simulink model "Bdot_control"  (R2023a)
settings: Solver=ode45  StartTime=0.0  StopTime=5830.0  RelTol=1e-3  EnableMultiTasking=on
libraries: aausat3_lib x6
settings Model: Creator=kasperv  LastModifiedBy=jacobel-omar
settings SolverCC: AlgebraicLoopSolver=TrustRegion
settings DataIOCC: LimitDataPoints=on  SaveFormat=Array  SignalLoggingSaveFormat=ModelDataLogs  ReturnWorkspaceOutputs=off
settings OptimizationCC: ExpressionDepthLimit=2147483647  LifeSpan=inf
settings DebuggingCC: UnderspecifiedInitializationDetection=Classic  MergeDetectMultiDrivingBlocksExec=none  SolverPrmCheckMsg=warning  FcnCallInpInsideContextMsg=warning  UnconnectedInputMsg=warning  UnconnectedOutputMsg=warning  UnconnectedLineMsg=warning  StateNameClashWarn=warning  SFUnexpectedBacktrackingDiag=warning  SFNoUnconditionalDefaultTransitionDiag=warning  SFExecutionAtInitializationDiag=none  ArithmeticOperatorsInVariantConditions=warning
settings HardwareCC: ProdBitPerPointer=32  ProdBitPerSizeT=32  ProdBitPerPtrDiffT=32  ProdLargestAtomicFloat=None  ProdIntDivRoundTo=Undefined  ProdEndianess=Unspecified  ProdWordSize=32  ProdHWDeviceType=32-bit Generic
settings ModelReferenceCC: EnableRefExpFcnMdlSchedulingChecks=on  PropagateSignalLabelsOutOfModel=off
settings SFSimCC: SimUseLocalCustomCode=off  CustomCodeUndefinedFunction=UseInterfaceOnly
settings RTWCC: RTWUseLocalCustomCode=off
settings CodeAppCC: StateflowObjectComments=on
settings GRTTargetCC: TargetLangStandard=C89/C90 (ANSI)  CombineOutputUpdateFcns=off  GRTInterface=on
settings ConfigComp: CovMetricSettings=dw  CovSaveCumulativeToWorkspaceVar=on  CovSaveSingleToWorkspaceVar=on  CovExternalEMLEnable=off

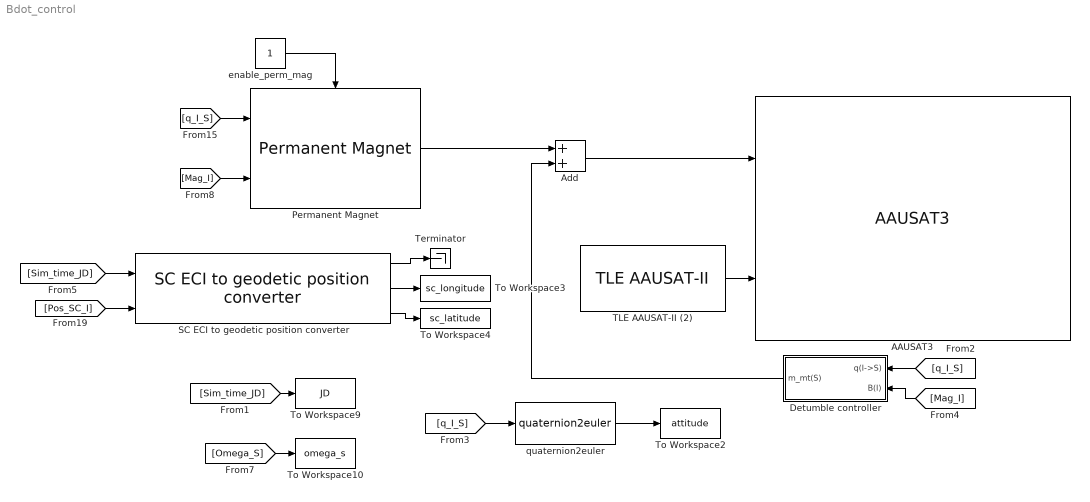
== system Bdot_control ==
  AAUSAT3 : aausat3_lib/AAUSAT3  r_com_s=[0.0493,0.0972,0.0549]  sat_temp_start=293.15  mass_sc=0.7924  Dim=[0.1,0.2,0.1]  inertia_c=[0.001653238447870,0.003461850559345,0.003630565819922]  init_jd=0  q_s_c=|  q_init_I_S=[0 0 0 1]  w_init_s=[0.17,0.17,0.17]  Cd=2  rho=5e-14  solar_m_flux=4.5565e-6  solar_absorb_coeff=1.5  theta_e=65  refldata=load('lib/AlbedoToolbox-1.0/refl_data/2005/ga050101-051231')  redfac=1  Ts=1  enable_sensor_emulation=on  enable_env_disturbance=off
      | [-0.192277302954935 -0.188661962989721 -0.681874874736906 0.680060848521491
      | ]
      link override Orbit and Magnetic field models1: reflectivity_enabled=off
      settings: SourceProductName=AAUSAT3
  Add : Sum
  Detumble controller : Subsystem  mask{C_cont=11000, w_c=0.7}
      mask prompts: C_cont "B-dot continous gain"; w_c "B-dot filter cut-off frequency"
  Permanent Magnet : aausat3_lib/Actuator Emulation/Permanent Magnet  mag_moment=0.0030
      settings: SourceProductName=AAUSAT3
  SC ECI to geodetic position converter : aausat3_lib/Other Model Utilities/SC ECI to geodetic position converter
      settings: SourceProductName=AAUSAT3
  TLE AAUSAT-II (2) : aausat3_lib/Orbit and Ephemeris/TLE AAUSAT-II  satname='AAUSAT-II'  JulianDay=09321.69542252  xndt2o=0.00000555  xndd6o=0.0  bstar=.76898e-4  xincl=97.9251  xnodeo=24.1597  eo=0.0014245  omegao=254.1774  xmo=105.7862  xno=14.81823818  ts=1
      settings: SourceProductName=AAUSAT3
  Terminator : Terminator
  To Workspace10 : ToWorkspace  VariableName=omega_s  SampleTime=-1
  To Workspace2 : ToWorkspace  VariableName=attitude  SampleTime=-1
  To Workspace3 : ToWorkspace  VariableName=sc_longitude  SampleTime=1
  To Workspace4 : ToWorkspace  VariableName=sc_latitude  SampleTime=1
  To Workspace9 : ToWorkspace  VariableName=JD  SampleTime=-1
  enable_perm_mag : Constant
  quaternion2euler : aausat3_lib/Math Utilities/Quaternion operations/quaternion2euler  SystemSampleTime=-1  VariantActivationTime=update diagram  Latency=0  AutoFrameSizeCalculation=off
      settings: SourceProductName=AAUSAT3
  wires:
  TLE AAUSAT-II (2)/1 -> AAUSAT3/2
  [Sim_time_JD] -> To Workspace9/1
  [Omega_S] -> To Workspace10/1
  [q_I_S] -> quaternion2euler/1
  quaternion2euler/1 -> To Workspace2/1
  [Sim_time_JD] -> SC ECI to geodetic position converter/1
  [Pos_SC_I] -> SC ECI to geodetic position converter/2
  SC ECI to geodetic position converter/1 -> Terminator/1
  SC ECI to geodetic position converter/2 -> To Workspace3/1
  SC ECI to geodetic position converter/3 -> To Workspace4/1
  [q_I_S] -> Permanent Magnet/1
  [Mag_I] -> Permanent Magnet/2
  enable_perm_mag/1 -> Permanent Magnet/Enable
  Permanent Magnet/1 -> Add/1
  Add/1 -> AAUSAT3/1
  [q_I_S] -> Detumble controller/1(q(I->S))
  [Mag_I] -> Detumble controller/2(B(I))
  Detumble controller/1(m_mt(S)) -> Add/2

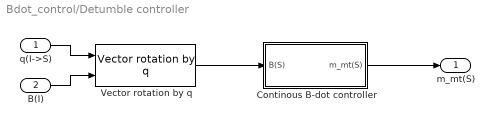
== system Bdot_control/Detumble controller ==
  q(I->S) : Inport
  B(I) : Inport  Port=2
  Continous B-dot controller : Subsystem
  Vector rotation by q : aausat3_lib/Math Utilities/Quaternion operations/Vector rotation by q  SystemSampleTime=-1  VariantActivationTime=update diagram  Latency=0  AutoFrameSizeCalculation=off
      settings: SourceProductName=AAUSAT3
  m_mt(S) : Outport
  wires:
  B(I)/1 -> Vector rotation by q/2
  q(I->S)/1 -> Vector rotation by q/1
  Vector rotation by q/1 -> Continous B-dot controller/1(B(S))
  Continous B-dot controller/1(m_mt(S)) -> m_mt(S)/1

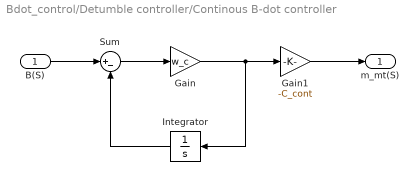
== system Bdot_control/Detumble controller/Continous B-dot controller ==
  B(S) : Inport
  Gain : Gain  Gain=w_c
  Gain1 : Gain  Gain=-C_cont
  Integrator : Integrator
  Sum : Sum  Inputs=|+-
  m_mt(S) : Outport
  wires:
  Gain1/1 -> m_mt(S)/1
  Integrator/1 -> Sum/2
  Gain/1 -> Integrator/1, Gain1/1
  Sum/1 -> Gain/1
  B(S)/1 -> Sum/1
